simulink model "Battery"  (R2023a)
settings: Solver=VariableStepAuto  StartTime=0.0  StopTime=24*3600  RelTol=1e-3
libraries: simulink x1
settings Model: PacingRate=1000  Creator=drdev  LastModifiedBy=alexa

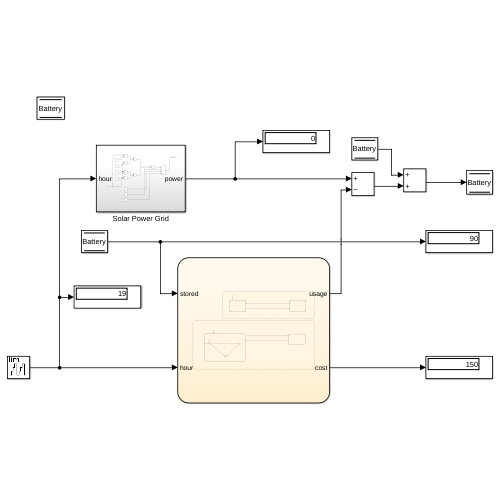
[thumbnail: Simulink's stored preview of the top-level diagram]
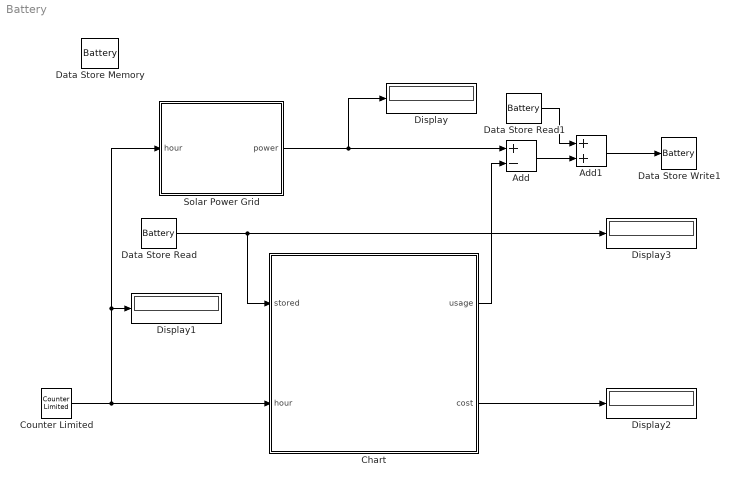
== system Battery ==
  Add : Sum  Inputs=+-
  Add1 : Sum
  Chart : Stateflow chart  TreatAsAtomicUnit=on
  Counter Limited : simulink/Sources/Counter Limited  uplimit=23  tsamp=-1
  Data Store Memory : DataStoreMemory  DataStoreName=Battery  WriteAfterWriteMsg=warning  ShowAdditionalParam=off
  Data Store Read : DataStoreRead  DataStoreName=Battery  IndexOptions=Index vector (dialog)  Indices=1  OutputSizes=1
  Data Store Read1 : DataStoreRead  DataStoreName=Battery  IndexOptions=Index vector (dialog)  Indices=1  OutputSizes=1
  Data Store Write1 : DataStoreWrite  DataStoreName=Battery  IndexOptions=Index vector (dialog)  Indices=1  OutputSizes=1
  Display{,1..3} (4 alike) : Display
  Solar Power Grid : Subsystem
  wires:
  Counter Limited/1 -> Solar Power Grid/1(hour), Display1/1, Chart/2(hour)
  Chart/1(usage) -> Add/2
  Solar Power Grid/1(power) -> Add/1, Display/1
  Add/1 -> Add1/2
  Data Store Read/1 -> Display3/1, Chart/1(stored)
  Chart/2(cost) -> Display2/1
  Add1/1 -> Data Store Write1/1
  Data Store Read1/1 -> Add1/1

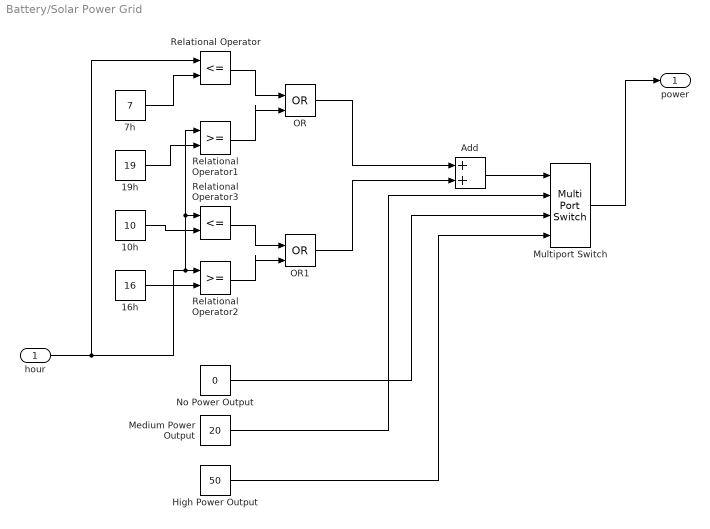
== system Battery/Solar Power Grid ==
  hour : Inport
  10h : Constant  Value=10
  16h : Constant  Value=16
  19h : Constant  Value=19
  7h : Constant  Value=7
  Add : Sum  InputSameDT=on
  High Power Output : Constant  Value=50
  Medium Power Output : Constant  Value=20
  Multiport Switch : MultiPortSwitch  DataPortOrder=Specify indices  DataPortIndices={1,2,0}  SaturateOnIntegerOverflow=off  InputSameDT=off
  No Power Output : Constant  Value=0
  OR : Logic  Operator=OR  IconShape=distinctive  AllPortsSameDT=off  OutDataTypeStr=boolean
  OR1 : Logic  Operator=OR  IconShape=distinctive  AllPortsSameDT=off  OutDataTypeStr=boolean
  Relational Operator : RelationalOperator  Operator=<=  OutDataTypeStr=boolean  RndMeth=Simplest  InputSameDT=off
  Relational Operator1 : RelationalOperator  OutDataTypeStr=boolean  RndMeth=Simplest  InputSameDT=off
  Relational Operator2 : RelationalOperator  OutDataTypeStr=boolean  RndMeth=Simplest  InputSameDT=off
  Relational Operator3 : RelationalOperator  Operator=<=  OutDataTypeStr=boolean  RndMeth=Simplest  InputSameDT=off
  power : Outport  OutMin=0  OutMax=0
  wires:
  hour/1 -> Relational Operator1/1, Relational Operator3/1, Relational Operator2/1, Relational Operator/1
  Multiport Switch/1 -> power/1
  7h/1 -> Relational Operator/2
  19h/1 -> Relational Operator1/2
  Relational Operator/1 -> OR/1
  Relational Operator1/1 -> OR/2
  No Power Output/1 -> Multiport Switch/3
  Medium Power Output/1 -> Multiport Switch/2
  High Power Output/1 -> Multiport Switch/4
  OR/1 -> Add/1
  16h/1 -> Relational Operator2/2
  OR1/1 -> Add/2
  Relational Operator2/1 -> OR1/2
  Relational Operator3/1 -> OR1/1
  10h/1 -> Relational Operator3/2
  Add/1 -> Multiport Switch/1

== stateflow chart Battery/Chart ==
  state usageTime [parallel]
    settings: executionOrder=1
    state offPeak
    state peak
    (default) -> offPeak
    peak -> offPeak : [hour >=18 || hour < 6]
    offPeak -> peak : [hour >= 6 && hour < 18]
  state usageType [parallel]
    settings: executionOrder=2
    state useGrid
      (default) -> (junction 19)
      (junction 19) -> (junction 22) [order 1] : [in(usageTime.peak)]
      useGrid -> (junction 19) [order 1]
      (junction 22) -> (junction 26) : {cost = cost + 15;}
      (junction 19) -> (junction 26) [order 2] : {cost = cost + 10;}
    state useBattery
      entry:
      usage = 40;
      exit:
      usage = 0;
    (default) -> useGrid : {cost = 0;}
    useGrid -> useBattery [order 1] : [stored > 80]
    useBattery -> useGrid : [stored < 40]
  data: stored input; usage output; hour input; cost output
